simulink model "requriment_3"  (R2021a)
settings: Solver=FixedStepDiscrete  StartTime=0.0  StopTime=50  FixedStep=1  RelTol=1e-3
undefined symbols (not defined in the file): sigbuilder_block
libraries: simulink x3
settings Model: Creator=Admin  LastModifiedBy=Rahul
settings SolverCC: AlgebraicLoopSolver=TrustRegion
settings DataIOCC: InspectSignalLogs=on  SignalLoggingName=sil_out  LoggingToFile=on  LoggingFileName=sil_out.mat
settings OptimizationCC: DefaultParameterBehavior=Inlined  UseDivisionForNetSlopeComputation=on  EnhancedBackFolding=on  PassReuseOutputArgsAs=Individual arguments  OptimizeBlockOrder=speed  DifferentSizesBufferReuse=on  OptimizationCustomize=off  EfficientTunableParamExpr=on
settings DebuggingCC: SignalInfNanChecking=error  ParameterTunabilityLossMsg=error  UniqueDataStoreMsg=error  AssertControl=DisableAll  StrictBusMsg=ErrorOnBusTreatedAsVector  SFUndirectedBroadcastEventsDiag=error  SFMachineParentedDataDiag=warning
settings SFSimCC: CompileTimeRecursionLimit=0  EnableRuntimeRecursion=off  MATLABDynamicMemAlloc=off  CustomCodeUndefinedFunction=UseInterfaceOnly
settings RTWCC: SystemTargetFile=ert.tlc  TemplateMakefile=ert_default_tmf  GenerateReport=on  IncludeHyperlinkInReport=on  LaunchReport=on  PortableWordSizes=on  GenerateTraceInfo=on  GenerateTraceReport=on  GenerateTraceReportSl=on  GenerateTraceReportSf=on  GenerateTraceReportEml=on
settings CodeAppCC: ForceParamTrailComments=on  IgnoreCustomStorageClasses=off  OperatorAnnotations=on  SimulinkDataObjDesc=on  SFDataObjDesc=on  MATLABFcnDesc=on  InsertBlockDesc=on
settings ERTTargetCC: TargetLangStandard=C99 (ISO)  UtilityFuncGeneration=Shared location  GenerateSampleERTMain=on  SupportNonFinite=off  ParenthesesLevel=Maximum  CastingMode=Standards  GenerateSharedConstants=off  InlinedParameterPlacement=NonHierarchical  ERTCustomFileTemplate=example_file_process.tlc  EnableSignedLeftShifts=off  EnableSignedRightShifts=off
settings ConfigComp: CovEnable=on  RecordCoverage=on  CovMetricSettings=dcmwe  CovModelRefEnable=on  DVMode=DesignErrorDetection  DVTestSuiteOptimization=Auto  DVDetectOutOfBounds=on  DVRebuildModelRepresentation=Always

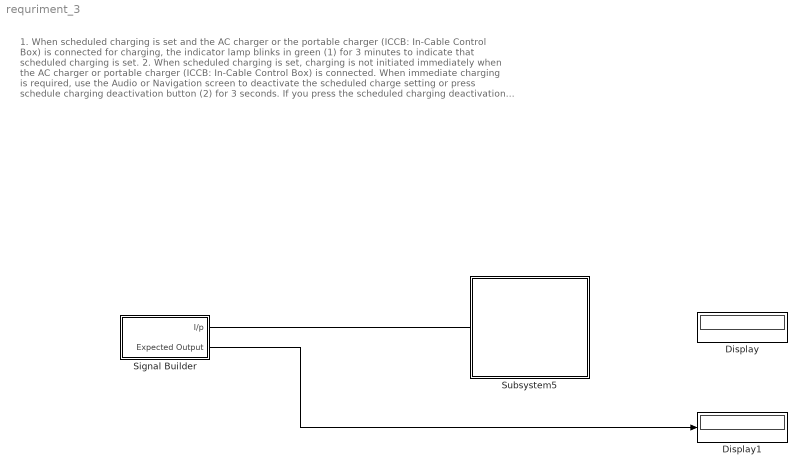
== system requriment_3 ==
  note: 1. When scheduled charging is set and the AC charger or the portable charger (ICCB: In-Cable Control Box) is connected for charging,
      | the indicator lamp blinks in green (1) for 3 minutes to indicate that scheduled charging is set.
      | 2. When scheduled charging is set,
      | charging is not initiated immediately when the AC charger or portable charger (ICCB: In-Cable Control Box) is connected. When immediate charging is required,
      | use the Audio or Navigation screen to deactivate the scheduled charge setting or press schedule charging deactivation button (2) for 3 seconds.
      | If you press the scheduled charging deactivation button (2) to immediately charge the battery,
      | charging must be initiated 3 minutes after the charging cable has been connected. When you press the scheduled charging deactivation button (2) for immediate charging, the scheduled charge setting
  Display : Display
  Display1 : Display
  Signal Builder : Subsystem  Tag=STV Subsys  LoadFcn=sigbuilder_block('load');  StartFcn=sigbuilder_block('start');  StopFcn=sigbuilder_block('stop');  ClipboardFcn=sigbuilder_block('clipboard');  mask(Sigbuilder block){tuvar=[0:10]}
      mask help: Simulink:masks:SigbuilderBlock_MD
      mask init:
      | if ~strcmp(get_param(bdroot(gcbh),'SimulationStatus'),'stopped') tuvar = sigbuilder_block('maskInit'); end
      settings: CopyFcn=sigbuilder_block('copy');  DeleteFcn=sigbuilder_block('delete');  ModelCloseFcn=sigbuilder_block('modelClose');  PreSaveFcn=sigbuilder_block('preSave');  PauseFcn=sigbuilder_block('pause');  ContinueFcn=sigbuilder_block('continue');  NameChangeFcn=sigbuilder_block('namechange');  OpenFcn=sigbuilder_block('open',[404 117.5 550.5 362.5 ]);  CloseFcn=sigbuilder_block('close');
      mask Display: plot(0, 0, 100, 100,[2, 2, 32, 32, 2], [68, 8, 8, 68, 68],[32, 2], [38, 38], [32, 19, 2],[53, 60, 44], [32, 17, 17, 2],[16, 16, 31, 31]);txt = getActiveGroup(gcbh);text(2, 100, txt,'verticalAlignment', 'top');
  Subsystem5 : Subsystem  TreatAsAtomicUnit=on
  wires:
  ? -> Display/1
  Signal Builder/1(I/p) -> ?
  Signal Builder/2(Expected Output) -> Display1/1

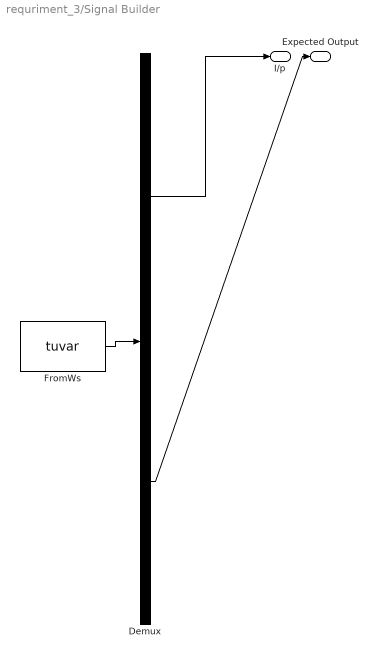
== system requriment_3/Signal Builder ==
  Demux : Demux  Tag=STV Demux  Outputs=2
      settings: DisplayOption=none
  FromWs : FromWorkspace  Tag=STV FromWs  VariableName=tuvar
      SigBuilderData=|
      | common.afterFinalStr = 'Extrapolate'
      | common.sampleTime = 0
      | dataSet.timeRange = [0 9]
      | dataSet.name = 'Sheet1'
      | sbobj.Name = 'Signal Builder'
      | sbobj.Groups.Name = 'Sheet1'
      | sbobj.Groups.Signals(1).Name = 'I/p'
      | sbobj.Groups.Signals(1).XData = [0 1 2 3 4 5 6 7 8 9]
      | sbobj.Groups.Signals(1).YData = [5 10 15 4 2 10 20 30 40 15]
      | sbobj.Groups.Signals(2).Name = 'Expected Output'
      | sbobj.Groups.Signals(2).XData = [0 1 2 3 4 5 6 7 8 9]
      | sbobj.Groups.Signals(2).YData = [1 0 -1 1 1 0 -1 1 1 -1]
      | sbobj.Groups.TimeRange = [0 9]
  I/p : Outport  Tag=STV Outport  VectorParamsAs1DForOutWhenUnconnected=off
  Expected Output : Outport  Tag=STV Outport  Port=2  VectorParamsAs1DForOutWhenUnconnected=off
  wires:
  Demux/1 -> I/p/1
  FromWs/1 -> Demux/1
  Demux/2 -> Expected Output/1

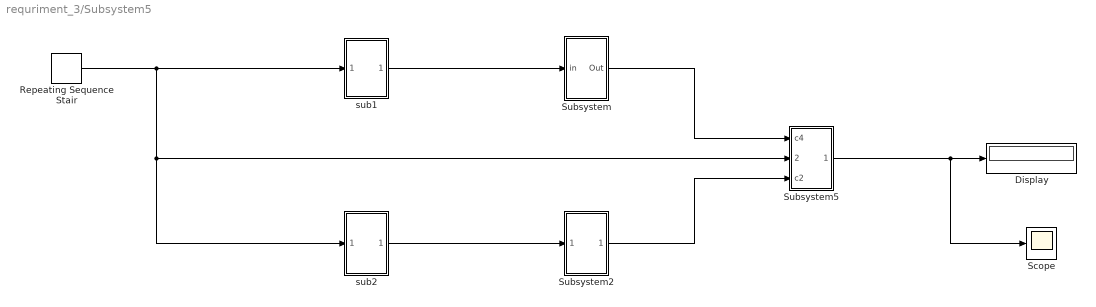
== system requriment_3/Subsystem5 ==
  Display : Display
  Repeating Sequence Stair : simulink/Sources/Repeating Sequence Stair  OutValues=[1 1 1 1 1 1 1 1 1 1 1 0 0 0 0 0]  tsamp=-1  OutMin=[]  OutMax=[]  OutDataTypeStr=double  OutputDataTypeScalingMode=double  OutDataType=fixdt(0,8)  ConRadixGroup=Best Precision: Vector-wise  OutScaling=2^-12
  Scope : Scope
  Subsystem : Subsystem
  Subsystem2 : Subsystem
  Subsystem5 : Subsystem
  sub1 : Subsystem
      settings: PermitHierarchicalResolution=None
  sub2 : Subsystem
  wires:
  Repeating Sequence Stair/1 -> sub1/1(in2), Subsystem5/2(In2), sub2/1(in1)
  sub2/1(out) -> Subsystem2/1(In1)
  sub1/1(out) -> Subsystem/1(in)
  Subsystem/1(Out) -> Subsystem5/1(c4)
  Subsystem2/1(Out1) -> Subsystem5/3(c2)
  Subsystem5/1(Out1) -> Scope/1, Display/1

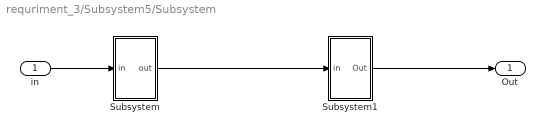
== system requriment_3/Subsystem5/Subsystem ==
  in : Inport
  Subsystem : Subsystem
  Subsystem1 : Subsystem
  Out : Outport  VectorParamsAs1DForOutWhenUnconnected=off
  wires:
  Subsystem/1(out) -> Subsystem1/1(in)
  Subsystem1/1(Out) -> Out/1
  in/1 -> Subsystem/1(in)

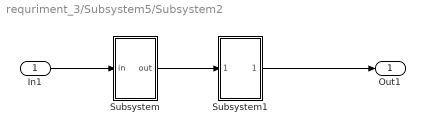
== system requriment_3/Subsystem5/Subsystem2 ==
  In1 : Inport
  Subsystem : Subsystem
  Subsystem1 : Subsystem
  Out1 : Outport  VectorParamsAs1DForOutWhenUnconnected=off
  wires:
  Subsystem1/1(out) -> Out1/1
  Subsystem/1(out) -> Subsystem1/1(In1)
  In1/1 -> Subsystem/1(in)

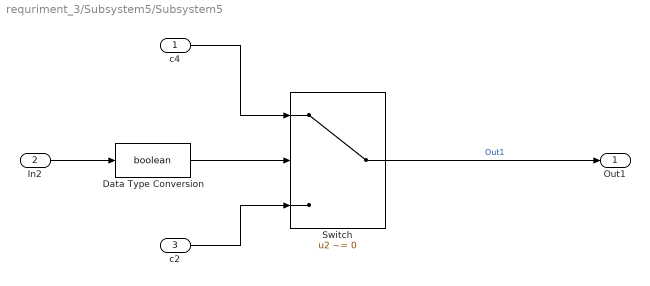
== system requriment_3/Subsystem5/Subsystem5 ==
  c4 : Inport
  In2 : Inport  Port=2
  c2 : Inport  Port=3
  Data Type Conversion : DataTypeConversion  OutDataTypeStr=boolean
  Switch : Switch  Criteria=u2 ~= 0  OutDataTypeStr=boolean
  Out1 : Outport  VectorParamsAs1DForOutWhenUnconnected=off
  wires:
  Switch/1 -> Out1/1  "Out1"
  c4/1 -> Switch/1
  c2/1 -> Switch/3
  In2/1 -> Data Type Conversion/1
  Data Type Conversion/1 -> Switch/2

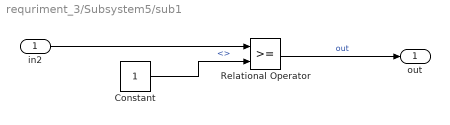
== system requriment_3/Subsystem5/sub1 ==
  in2 : Inport
  Constant : Constant
  Relational Operator : RelationalOperator  OutDataTypeStr=boolean  RndMeth=Simplest
  out : Outport  VectorParamsAs1DForOutWhenUnconnected=off
  wires:
  in2/1 -> Relational Operator/1
  Constant/1 -> Relational Operator/2  "<>"
  Relational Operator/1 -> out/1  "out"

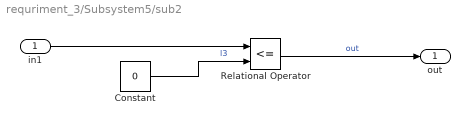
== system requriment_3/Subsystem5/sub2 ==
  in1 : Inport
  Constant : Constant  Value=0
  Relational Operator : RelationalOperator  Operator=<=  OutDataTypeStr=boolean  RndMeth=Simplest
  out : Outport  VectorParamsAs1DForOutWhenUnconnected=off
  wires:
  Relational Operator/1 -> out/1  "out"
  Constant/1 -> Relational Operator/2  "l3"
  in1/1 -> Relational Operator/1

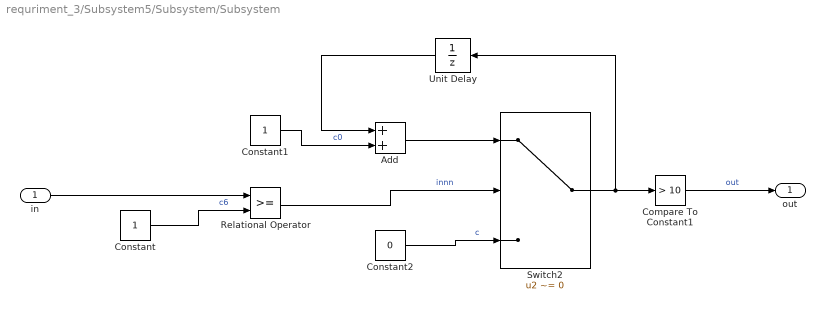
== system requriment_3/Subsystem5/Subsystem/Subsystem ==
  in : Inport
  Add : Sum
  Compare To Constant1 : simulink/Logic and Bit Operations/Compare To Constant  relop=>  const=10  OutDataTypeStr=boolean
  Constant : Constant
  Constant1 : Constant
  Constant2 : Constant  Value=0
  Relational Operator : RelationalOperator  OutDataTypeStr=boolean  RndMeth=Simplest
  Switch2 : Switch  Criteria=u2 ~= 0
  Unit Delay : UnitDelay  SampleTime=-1  HasFrameUpgradeWarning=on
  out : Outport  VectorParamsAs1DForOutWhenUnconnected=off
  wires:
  Compare To Constant1/1 -> out/1  "out"
  Constant/1 -> Relational Operator/2  "c6"
  Unit Delay/1 -> Add/1
  Relational Operator/1 -> Switch2/2  "innn"
  Add/1 -> Switch2/1
  Switch2/1 -> Unit Delay/1, Compare To Constant1/1
  Constant2/1 -> Switch2/3  "c"
  in/1 -> Relational Operator/1
  Constant1/1 -> Add/2  "c0"

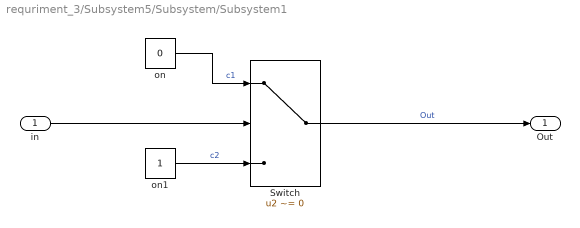
== system requriment_3/Subsystem5/Subsystem/Subsystem1 ==
  in : Inport
  Switch : Switch  Criteria=u2 ~= 0  OutDataTypeStr=boolean
  on : Constant  Value=0  OutDataTypeStr=boolean
  on1 : Constant
  Out : Outport  VectorParamsAs1DForOutWhenUnconnected=off
  wires:
  Switch/1 -> Out/1  "Out"
  in/1 -> Switch/2
  on1/1 -> Switch/3  "c2"
  on/1 -> Switch/1  "c1"

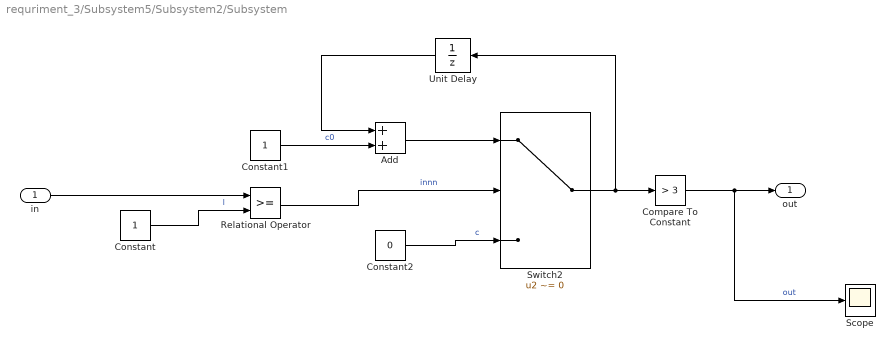
== system requriment_3/Subsystem5/Subsystem2/Subsystem ==
  in : Inport
  Add : Sum
  Compare To Constant : simulink/Logic and Bit Operations/Compare To Constant  relop=>  const=3  OutDataTypeStr=boolean
  Constant : Constant
  Constant1 : Constant
  Constant2 : Constant  Value=0
  Relational Operator : RelationalOperator  OutDataTypeStr=boolean  RndMeth=Simplest
  Scope : Scope
  Switch2 : Switch  Criteria=u2 ~= 0
  Unit Delay : UnitDelay  SampleTime=-1  HasFrameUpgradeWarning=on
  out : Outport  VectorParamsAs1DForOutWhenUnconnected=off
  wires:
  Add/1 -> Switch2/1
  in/1 -> Relational Operator/1
  Switch2/1 -> Unit Delay/1, Compare To Constant/1
  Relational Operator/1 -> Switch2/2  "innn"
  Compare To Constant/1 -> Scope/1, out/1  "out"
  Unit Delay/1 -> Add/1
  Constant2/1 -> Switch2/3  "c"
  Constant1/1 -> Add/2  "c0"
  Constant/1 -> Relational Operator/2  "l"

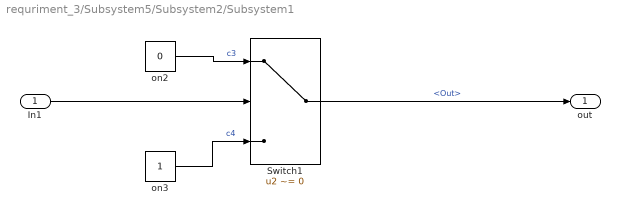
== system requriment_3/Subsystem5/Subsystem2/Subsystem1 ==
  In1 : Inport
  Switch1 : Switch  Criteria=u2 ~= 0
  on2 : Constant  Value=0  OutDataTypeStr=boolean
  on3 : Constant
  out : Outport  VectorParamsAs1DForOutWhenUnconnected=off
  wires:
  Switch1/1 -> out/1  "<Out>"
  In1/1 -> Switch1/2
  on2/1 -> Switch1/1  "c3"
  on3/1 -> Switch1/3  "c4"
